simulink model "TrafficLightNegotiationTestBench"  (R2022b)
settings: Solver=ode23tb  StartTime=0.0  StopTime=scenario.StopTime  FixedStep=0.001  RelTol=1e-8  EnableMultiTasking=on
model workspace (MAT data in the model file):
  green = 'green'
values from neighbouring files (symbols this model uses):
  intersectionInfo = evalin('base', 'intersectionInfo')    [HelperTrafficLightNegotiationVisualization.m]
undefined symbols (not defined in the file or in its folder): Curvature, CurvatureDerivative, driving, HeadingAngle, LateralOffset, Left, M, matlabshared, N, referencePathInfo, Right, Strength, Ts, v_set
libraries: drivingscenarioandsensors x4, trackingutilitieslib x1, drivinglib x1
CloseFcn:
  | helperSLTrafficLightNegotiationCleanUp
settings Model: Creator=The MathWorks, Inc.  LastModifiedBy=sangm
settings SolverCC: ZeroCrossAlgorithm=Adaptive  AlgebraicLoopSolver=TrustRegion  PositivePriorityOrder=on  AutoInsertRateTranBlk=on  InsertRTBMode=Always  DecoupledContinuousIntegration=on  MinimalZcImpactIntegration=on  MaxZcPerStep=1
settings DataIOCC: SaveOutput=off  SaveTime=off  ReturnWorkspaceOutputs=off
settings DebuggingCC: MaskedZcDiagnostic=none  IgnoredZcDiagnostic=none  ParameterPrecisionLossMsg=none  UnconnectedInputMsg=warning  UnconnectedOutputMsg=warning  UnconnectedLineMsg=warning  PregeneratedLibrarySubsystemCodeDiagnostic=none  SFMachineParentedDataDiag=warning  ArithmeticOperatorsInVariantConditions=warning
settings HardwareCC: ProdLongLongMode=on
settings ModelReferenceCC: EnableRefExpFcnMdlSchedulingChecks=on
settings SFSimCC: SimUseLocalCustomCode=off
settings RTWCC: GenerateReport=on  RTWUseLocalCustomCode=off  LaunchReport=on  DLArmComputeVersion=19.05
settings ConfigComp: CovScope=ReferencedModels  CovIncludeTopModel=off

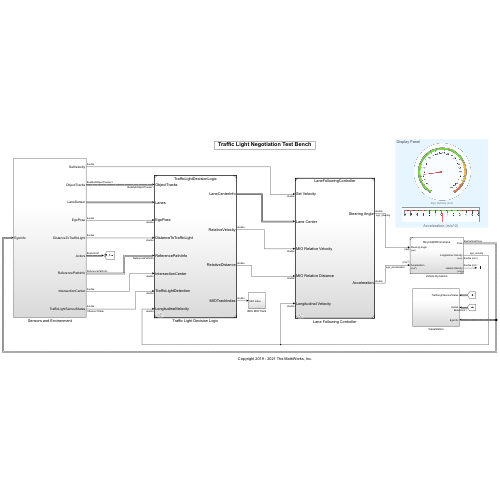
[thumbnail: Simulink's stored preview of the top-level diagram]
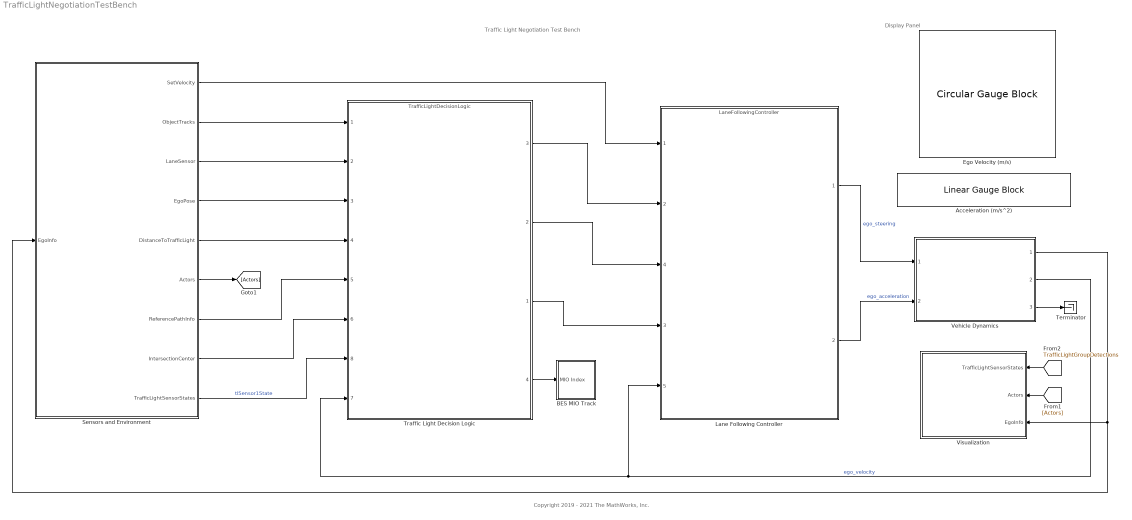
== system TrafficLightNegotiationTestBench ==
  note: Traffic Light Negotiation Test Bench
  note: Display Panel
  note: Copyright 2019 - 2021 The MathWorks, Inc.
  Acceleration (m/s^2) : LinearGaugeBlock  LabelPosition=Hide  ScaleMin=-6  ScaleMax=6
  BES MIO Track : Subsystem
  Ego Velocity (m/s) : CircularGaugeBlock  LabelPosition=Hide  ScaleMax=50
  Lane Following Controller : ModelReference  ModelNameDialog=LaneFollowingController.slx  SimulationMode=Normal  ModelReferenceVersion=6.1
      settings: PortSchema="{\"entries\":[{\"content\":{\"sides\":[{\"content\":{\"connectorIds\":[\"In1\",\"In2\",\"In4\",\"In3\",\"In5\"]},\"type\":\"ConnectorPlacement.EquallySpacedRectSide\",\"uuid\":\"258a64d3-b85d-4414-a7dd-6950fa9dc812\"},{\"content\":{\"connectorIds\":[\"Out1\",\"Out2\"],\"side\":\"RIGHT\"},\"type\":\"ConnectorPlacement.EquallySpacedRectSide\",\"uuid\":\"eccca8be-1d69-4bb6-a162-74a40ef18f77\"},{\"content\":{\"connectorIds\":[],\"side\":\"TOP\"},\"type\":\"ConnectorPlacement.EquallySpacedRectSide\",\"uuid\":\"90abafbb-8c91-4838-b7d8-ed3861625810\"}]},\"type\":\"ConnectorPlacement.EquallySpacedConnector\",\"uuid\":\"818faacf-e725-4a67-9fb9-d6eb3f95c5ad\"}],\"packageUris\":[\"http://schema.mathworks.com/mf0/Connector/R2020b\"],\"version\":\"1.0\"}"
  Sensors and Environment : Subsystem
  Terminator : Terminator
  Traffic Light Decision Logic : ModelReference  ModelNameDialog=TrafficLightDecisionLogic  SimulationMode=Normal  ModelReferenceVersion=5.1
      settings: PortSchema="{\"entries\":[{\"content\":{\"sides\":[{\"content\":{\"connectorIds\":[\"In1\",\"In2\",\"In3\",\"In4\",\"In5\",\"In6\",\"In8\",\"In7\"]},\"type\":\"ConnectorPlacement.EquallySpacedRectSide\",\"uuid\":\"580d7771-a392-489d-ba06-e0a23417c921\"},{\"content\":{\"connectorIds\":[\"Out3\",\"Out2\",\"Out1\",\"Out4\"],\"side\":\"RIGHT\"},\"type\":\"ConnectorPlacement.EquallySpacedRectSide\",\"uuid\":\"34dc41bc-0d5b-42f7-ac4d-a18cefff1604\"},{\"content\":{\"connectorIds\":[],\"side\":\"TOP\"},\"type\":\"ConnectorPlacement.EquallySpacedRectSide\",\"uuid\":\"c461dccf-2cc6-49a6-b643-9bb66a30f56a\"},{\"content\":{\"connectorIds\":[],\"side\":\"HIDDEN\"},\"type\":\"ConnectorPlacement.EquallySpacedRectSide\",\"uuid\":\"944284c5-f0c1-462b-8985-62524d7ec2e9\"}]},\"type\":\"ConnectorPlacement.EquallySpacedConnector\",\"uuid\":\"d6b87f41-7423-4eb9-8350-a9de1b3f3f98\"}],\"packageUris\":[\"http://schema.mathworks.com/mf0/Connector/R2020b\"],\"version\":\"1.0\"}"
  Vehicle Dynamics : Subsystem  ReferencedSubsystem=BicycleWithForceInput
  Visualization : Subsystem
  wires:
  Sensors and Environment/6(Actors) -> [Actors]
  Sensors and Environment/2(ObjectTracks) -> Traffic Light Decision Logic/1
  Lane Following Controller/2 -> Vehicle Dynamics/2  "ego_acceleration"
  Sensors and Environment/1(SetVelocity) -> Lane Following Controller/1
  Vehicle Dynamics/2 -> Traffic Light Decision Logic/7, Lane Following Controller/5  "ego_velocity"
  [TrafficLightGroupDetections] -> Visualization/1(TrafficLightSensorStates)
  Vehicle Dynamics/1 -> Sensors and Environment/1(EgoInfo), Visualization/3(EgoInfo)
  [Actors] -> Visualization/2(Actors)
  Sensors and Environment/4(EgoPose) -> Traffic Light Decision Logic/3
  Sensors and Environment/3(LaneSensor) -> Traffic Light Decision Logic/2
  Sensors and Environment/5(DistanceToTrafficLight) -> Traffic Light Decision Logic/4
  Sensors and Environment/7(ReferencePathInfo) -> Traffic Light Decision Logic/5
  Sensors and Environment/8(IntersectionCenter) -> Traffic Light Decision Logic/6
  Sensors and Environment/9(TrafficLightSensorStates) -> Traffic Light Decision Logic/8  "tlSensor1State"
  Traffic Light Decision Logic/3 -> Lane Following Controller/2
  Traffic Light Decision Logic/1 -> Lane Following Controller/3
  Traffic Light Decision Logic/2 -> Lane Following Controller/4
  Lane Following Controller/1 -> Vehicle Dynamics/1  "ego_steering"
  Traffic Light Decision Logic/4 -> BES MIO Track/1(MIO Index)
  Vehicle Dynamics/3 -> Terminator/1

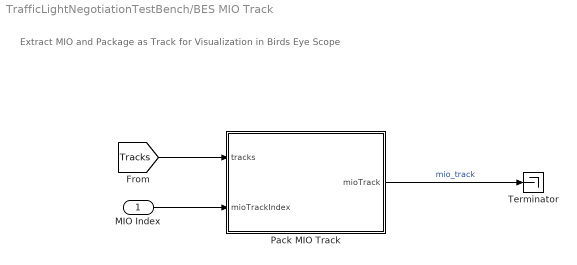
== system TrafficLightNegotiationTestBench/BES MIO Track ==
  note: Extract MIO and Package as Track for Visualization in Birds Eye Scope
  MIO Index : Inport
  Pack MIO Track : MATLAB Function  TreatAsAtomicUnit=on
  Terminator : Terminator
  wires:
  MIO Index/1 -> Pack MIO Track/2(mioTrackIndex)
  [Tracks] -> Pack MIO Track/1(tracks)
  Pack MIO Track/1(mioTrack) -> Terminator/1  "mio_track"

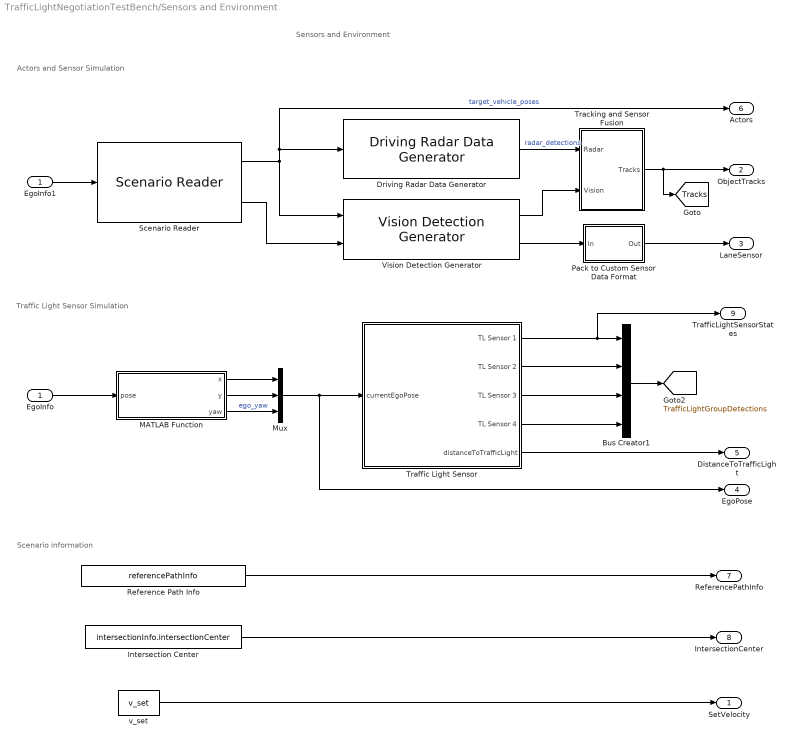
== system TrafficLightNegotiationTestBench/Sensors and Environment ==
  note: Scenario information
  note: Traffic Light Sensor Simulation
  note: Actors and Sensor Simulation
  note: Sensors and Environment
  EgoInfo : Inport
  Bus Creator1 : BusCreator  Inputs=4
  Driving Radar Data Generator : drivingscenarioandsensors/Driving Radar Data Generator  SensorIndex=2  UpdateRate=10  MountingLocation=[ 3.7, 0, 0.2 ]  MountingAngles=[0 0 0]  HasElevation=off  HasRangeRate=on  HasNoise=on  HasFalseAlarms=on  HasOcclusion=on  MaxNumReportsSource=Property  MaxNumReports=50  TargetReportFormat=Clustered detections  DetectionCoordinates=Body  TrackCoordinates=Body  BusNameSource=Property  BusName=BusRadar  AzimuthResolution=4  ElevationResolution=5  RangeResolution=2.5  RangeRateResolution=0.5  AzimuthBiasFraction=0.1  ElevationBiasFraction=0.1  RangeBiasFraction=0.05  RangeRateBiasFraction=0.05  FieldOfView=[ 20, 5 ]  RangeLimits=[ 0, 174 ]  RangeRateLimits=[ -100, 100 ]  DetectionProbability=0.9  FalseAlarmRate=1e-06  ReferenceRange=100  ReferenceRCS=0  CenterFrequency=77e9  FilterInitializationFcn=initcvekf  ConfirmationThreshold=[2 3]  DeletionThreshold=[5 5]  InitialSeedSource=Repeatable  InitialSeed=0  UsedSeed=matlabshared.tracking.internal.SimulinkUtilities.seedManager(gcb)  ProfilesSource=From Scenario Reader block  ProfilesParameters=driving.internal.ActorProfilesRadarParameters  ProfilesExpression=struct('ClassID',0,'Length',4.7,'Width',1.8,'Height',1.4,'OriginOffset',[-1.35 0 0],'RCSPattern',[10 10;10 10],'RCSAzimuthAngles',[-180 180],'RCSElevationAngles',[-90 90])
  EgoInfo1 : InportShadow
  Intersection Center : Constant  Value=intersectionInfo.intersectionCenter  SampleTime=Ts
      settings: AttributesFormatString=|
      | ------------------------------
      |    Value = %<Value>
  MATLAB Function : MATLAB Function  TreatAsAtomicUnit=on
  Mux : Mux  Inputs=3
  Pack to Custom Sensor Data Format : Subsystem
  Reference Path Info : Constant  Value=referencePathInfo  OutDataTypeStr=Bus: ReferencePathInfo  SampleTime=Ts
      settings: AttributesFormatString=|
      | --------------------------
      |   Value = %<Value>
  Scenario Reader : drivingscenarioandsensors/Scenario Reader  ScenarioSource=From workspace  ScenarioFileName=EgoVehicleGoesStraight.mat  ScenarioVariableName=scenario  OutputCoordinateSystem=Vehicle coordinates  EgoVehicleSource=Input port  EgoVehicleActorID=egoVehicle.ActorID  OrientVehiclesOnRoad=on  OutputEgoVehiclePose=off  OutputEgoVehicleState=off  SampleTime=Ts  LaneBoundaryOutput=All lane boundaries  LaneBoundaryDistance=0:0.5:60  LaneBoundaryLocation=Center of lane markings  BusNameSource=Auto  BusName=BusActors  BusNumActorsSource=Scenario  BusNumActors=100  BusName2Source=Auto  BusName2=BusLaneBoundaries  BusNumLaneBoundariesSource=Scenario  BusNumLaneBoundaries=10  BusName3Source=Auto  BusName3=BusEgoActor  BusName4Source=Auto  BusName4=BusEgoState  ShowCoordinateLabels=on  SimulateUsing=Interpreted execution
  Tracking and Sensor Fusion : Subsystem  TreatAsAtomicUnit=on  SystemSampleTime=Ts
      settings: RTWFileNameOpts=Use function name
  Traffic Light Sensor : Subsystem  mask{TrafficLightSensorModeSelection=Cycle, TrafficLightPosition=intersectionInfo.tlSensor1Position}
      mask prompts: TrafficLightSensorModeSelection "Traffic Light Sensor Mode:"; TrafficLightPosition "Traffic Light Position:"
      mask TypeOptions TrafficLightSensorModeSelection: Steady Green | Steady Red | Cycle
      mask TypeOptions TrafficLightPosition: TrafficLightPosition/Value
      mask DialogControl DescTextVar Prompt: Simulate a traffic light sensor.
  Vision Detection Generator : drivingscenarioandsensors/Vision Detection Generator  SensorIndex=1  DetectorOutput=Lanes and objects  UpdateInterval=0.1  LaneUpdateInterval=0.1  SensorLocation=[ 1.9, 0 ]  Height=1.1  Yaw=0  Pitch=1  Roll=0  BusNameSource=Property  BusName=BusVision  BusName2Source=Property  BusName2=BusLanes  MaxNumDetectionsSource=Property  MaxNumDetections=20  MaxNumLanesSource=Property  MaxNumLanes=2  DetectionCoordinates=Ego Cartesian  SimulateUsing=Interpreted execution  MaxRange=150  BoundingBoxAccuracy=5  ProcessNoiseIntensity=5  MaxSpeed=50  MaxAllowedOcclusion=0.5  MinObjectImageSize=[ 10, 10 ]  DetectionProbability=1  FalsePositivesPerImage=0  MinLaneImageSize=[ 20, 3 ]  LaneBoundaryAccuracy=3  HasNoise=off  InitialSeedSource=Repeatable  InitialSeed=0  UsedSeed=driving.internal.SimulinkUtilities.seedManager(gcb)  ActorProfilesSource=From Scenario Reader block  ActorProfilesParameters=driving.internal.ActorProfilesParameters  ActorProfilesExpression=struct( 'ClassID', 0, 'Length', 4.7, 'Width', 1.8, 'Height', 1.4, 'OriginOffset', [ -1.35, 0, 0 ] )  Intrinsics=driving.internal.cameraIntrinsics('FocalLength',[ 800,800 ])
  v_set : Constant  Value=v_set
  SetVelocity : Outport
  ObjectTracks : Outport  Port=2
  LaneSensor : Outport  Port=3  VectorParamsAs1DForOutWhenUnconnected=off
  EgoPose : Outport  Port=4
  DistanceToTrafficLight : Outport  Port=5
  Actors : Outport  Port=6
  ReferencePathInfo : Outport  Port=7
  IntersectionCenter : Outport  Port=8
  TrafficLightSensorStates : Outport  Port=9
  tag scope: Tracks=global, TrafficLightGroupDetections=global
  wires:
  Vision Detection Generator/2 -> Pack to Custom Sensor Data Format/1(In)
  Pack to Custom Sensor Data Format/1(Out) -> LaneSensor/1
  Scenario Reader/2 -> Vision Detection Generator/2
  Vision Detection Generator/1 -> Tracking and Sensor Fusion/2(Vision)
  Driving Radar Data Generator/1 -> Tracking and Sensor Fusion/1(Radar)  "radar_detections"
  EgoInfo/1 -> MATLAB Function/1(pose)
  MATLAB Function/3(yaw) -> Mux/3  "ego_yaw"
  MATLAB Function/2(y) -> Mux/2
  MATLAB Function/1(x) -> Mux/1
  Mux/1 -> EgoPose/1, Traffic Light Sensor/1(currentEgoPose)
  Tracking and Sensor Fusion/1(Tracks) -> [Tracks], ObjectTracks/1
  Scenario Reader/1 -> Driving Radar Data Generator/1, Actors/1, Vision Detection Generator/1  "target_vehicle_poses"
  EgoInfo1/1 -> Scenario Reader/1
  Traffic Light Sensor/5(distanceToTrafficLight) -> DistanceToTrafficLight/1
  Reference Path Info/1 -> ReferencePathInfo/1
  v_set/1 -> SetVelocity/1
  Intersection Center/1 -> IntersectionCenter/1
  Traffic Light Sensor/1(TL Sensor 1) -> TrafficLightSensorStates/1, Bus Creator1/1
  Traffic Light Sensor/2(TL Sensor 2) -> Bus Creator1/2
  Traffic Light Sensor/3(TL Sensor 3) -> Bus Creator1/3
  Traffic Light Sensor/4(TL Sensor 4) -> Bus Creator1/4
  Bus Creator1/1 -> [TrafficLightGroupDetections]

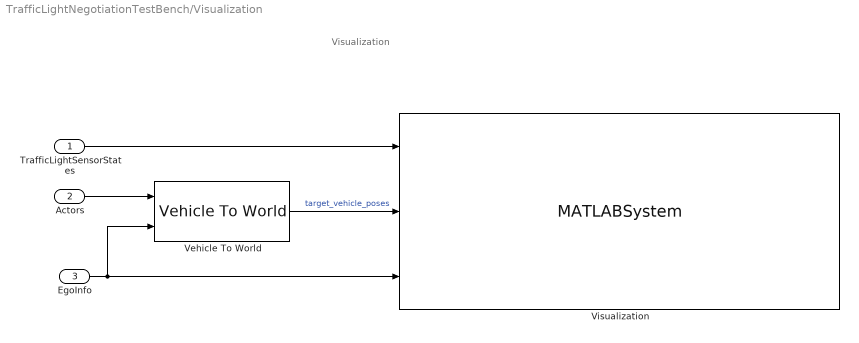
== system TrafficLightNegotiationTestBench/Visualization ==
  note: Visualization
  TrafficLightSensorStates : Inport
  Actors : Inport  Port=2
  EgoInfo : Inport  Port=3
  Vehicle To World : drivingscenarioandsensors/Vehicle To World  BusNameSource=Auto  BusName=BusVehicleToWorldActors  SimulateUsing=Interpreted execution
  Visualization : MATLABSystem  System=HelperTrafficLightNegotiationVisualization
      mask Type: HelperTrafficLightNegotiationVisualization
      mask Display:
      | disp('HelperTrafficLightNegotiationVisualization');
      | port_label('input',1,'TrafficLightSensorStates');
      | port_label('input',2,'TargetPoses');
      | port_label('input',3,'EgoInfo');
  wires:
  TrafficLightSensorStates/1 -> Visualization/1
  Actors/1 -> Vehicle To World/1
  EgoInfo/1 -> Vehicle To World/2, Visualization/3
  Vehicle To World/1 -> Visualization/2  "target_vehicle_poses"

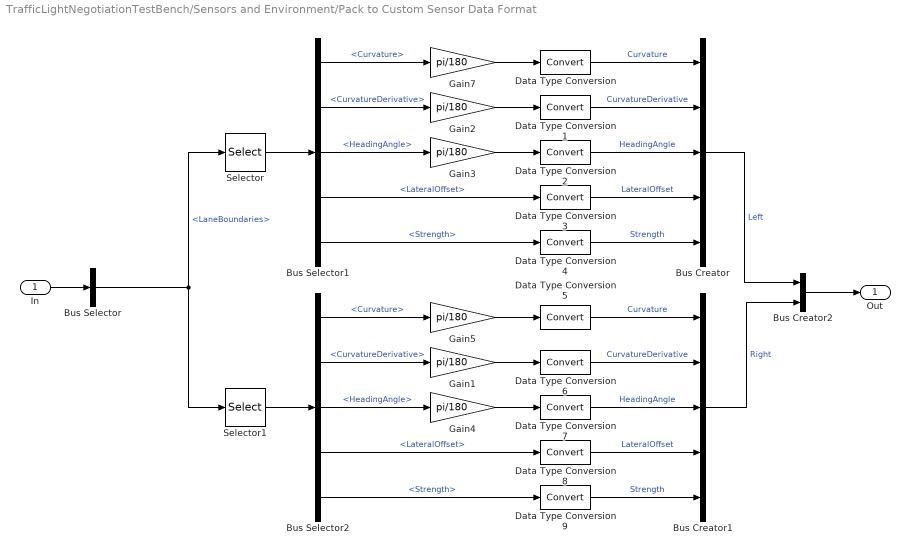
== system TrafficLightNegotiationTestBench/Sensors and Environment/Pack to Custom Sensor Data Format ==
  In : Inport
  Bus Creator : BusCreator  Inputs=Curvature,CurvatureDerivative,HeadingAngle,LateralOffset,Strength  OutDataTypeStr=Bus: LaneSensorBoundaries
  Bus Creator1 : BusCreator  Inputs=Curvature,CurvatureDerivative,HeadingAngle,LateralOffset,Strength  OutDataTypeStr=Bus: LaneSensorBoundaries
  Bus Creator2 : BusCreator  Inputs=Left,Right  OutDataTypeStr=Bus: LaneSensor
  Bus Selector : BusSelector  OutputSignals=LaneBoundaries
  Bus Selector1 : BusSelector  OutputSignals=Curvature,CurvatureDerivative,HeadingAngle,LateralOffset,Strength
  Bus Selector2 : BusSelector  OutputSignals=Curvature,CurvatureDerivative,HeadingAngle,LateralOffset,Strength
  Data Type Conversion{,1..9} (10 alike) : DataTypeConversion  SaturateOnIntegerOverflow=off  RndMeth=Floor
  Gain{1..5,7} (6 alike) : Gain  Gain=pi/180
  Selector : Selector  InputPortWidth=2  IndexOptions=Index vector (dialog)  Indices=1  OutputSizes=1
  Selector1 : Selector  InputPortWidth=2  IndexOptions=Index vector (dialog)  Indices=2  OutputSizes=1
  Out : Outport  VectorParamsAs1DForOutWhenUnconnected=off
  wires:
  In/1 -> Bus Selector/1
  Bus Selector/1 -> Selector/1, Selector1/1  "<LaneBoundaries>"
  Selector/1 -> Bus Selector1/1
  Bus Selector1/2 -> Gain2/1  "<CurvatureDerivative>"
  Bus Selector1/1 -> Gain7/1  "<Curvature>"
  Bus Selector1/3 -> Gain3/1  "<HeadingAngle>"
  Gain7/1 -> Data Type Conversion/1
  Gain2/1 -> Data Type Conversion1/1
  Gain3/1 -> Data Type Conversion2/1
  Bus Selector1/4 -> Data Type Conversion3/1  "<LateralOffset>"
  Bus Selector1/5 -> Data Type Conversion4/1  "<Strength>"
  Data Type Conversion/1 -> Bus Creator/1  "Curvature"
  Data Type Conversion1/1 -> Bus Creator/2  "CurvatureDerivative"
  Data Type Conversion2/1 -> Bus Creator/3  "HeadingAngle"
  Data Type Conversion3/1 -> Bus Creator/4  "LateralOffset"
  Data Type Conversion4/1 -> Bus Creator/5  "Strength"
  Data Type Conversion9/1 -> Bus Creator1/5  "Strength"
  Data Type Conversion6/1 -> Bus Creator1/2  "CurvatureDerivative"
  Data Type Conversion7/1 -> Bus Creator1/3  "HeadingAngle"
  Data Type Conversion8/1 -> Bus Creator1/4  "LateralOffset"
  Data Type Conversion5/1 -> Bus Creator1/1  "Curvature"
  Bus Selector2/1 -> Gain5/1  "<Curvature>"
  Selector1/1 -> Bus Selector2/1
  Bus Selector2/4 -> Data Type Conversion8/1  "<LateralOffset>"
  Bus Selector2/5 -> Data Type Conversion9/1  "<Strength>"
  Bus Selector2/2 -> Gain1/1  "<CurvatureDerivative>"
  Gain4/1 -> Data Type Conversion7/1
  Gain5/1 -> Data Type Conversion5/1
  Gain1/1 -> Data Type Conversion6/1
  Bus Selector2/3 -> Gain4/1  "<HeadingAngle>"
  Bus Creator2/1 -> Out/1
  Bus Creator/1 -> Bus Creator2/1  "Left"
  Bus Creator1/1 -> Bus Creator2/2  "Right"

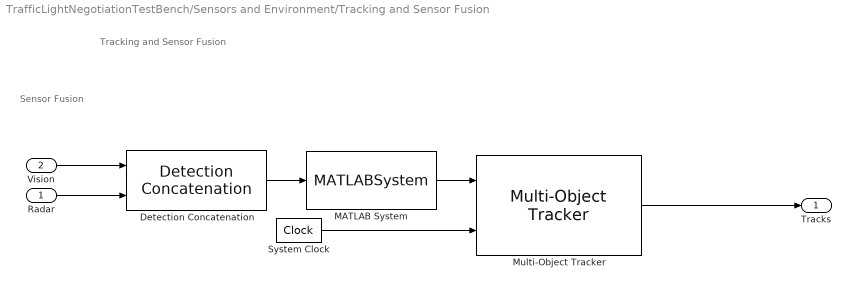
== system TrafficLightNegotiationTestBench/Sensors and Environment/Tracking and Sensor Fusion ==
  note: Tracking and Sensor Fusion
  note: Sensor Fusion
  Radar : Inport  PortDimensions=[1 1]  BusOutputAsStruct=on
  Vision : Inport  Port=2  PortDimensions=[1 1]  BusOutputAsStruct=on
  Detection Concatenation : trackingutilitieslib/Detection Concatenation  NumInputs=2  BusNameSource=Auto  BusName=BusDetectionConcatenation1  SimulateUsing=Interpreted execution
  MATLAB System : MATLABSystem  System=helperVehicleSize  VehicleSize=vehicleLength  BusNameSource=Auto  BusName=BusVehicleSizeDetections  SimulateUsing=Interpreted execution
      mask Type: helperVehicleSize
      mask Display:
      | disp('helperVehicleSize');
      | port_label('input',1,'In');
      | port_label('output',1,'Out');
  Multi-Object Tracker : drivinglib/Multi-Object Tracker  TrackerIndex=uint32( 0 )  FilterInitializationFcn=initcvekf  AssignmentThreshold=assignThresh  ConfirmationThreshold=[ M, N ]  DeletionThreshold=[ 5, 5 ]  MaxNumTracks=numTracks  MaxNumSensors=numSensors  OOSMHandling=Terminate  StateParametersSimulink=struct  HasStateParametersInput=off  TimeInputSource=Input port  HasCostMatrixInput=off  HasDetectableTrackIDsInput=off  BusNameSource=Property  BusName=BusMultiObjectTracker1  TentativeTracksOutputPort=off  AllTracksOutputPort=off  SimulateUsing=Interpreted execution
  System Clock : DigitalClock  SampleTime=-1
  Tracks : Outport  PortDimensions=[1 1]  VectorParamsAs1DForOutWhenUnconnected=off  BusOutputAsStruct=on
  wires:
  System Clock/1 -> Multi-Object Tracker/2
  Vision/1 -> Detection Concatenation/1
  Radar/1 -> Detection Concatenation/2
  Multi-Object Tracker/1 -> Tracks/1
  Detection Concatenation/1 -> MATLAB System/1
  MATLAB System/1 -> Multi-Object Tracker/1

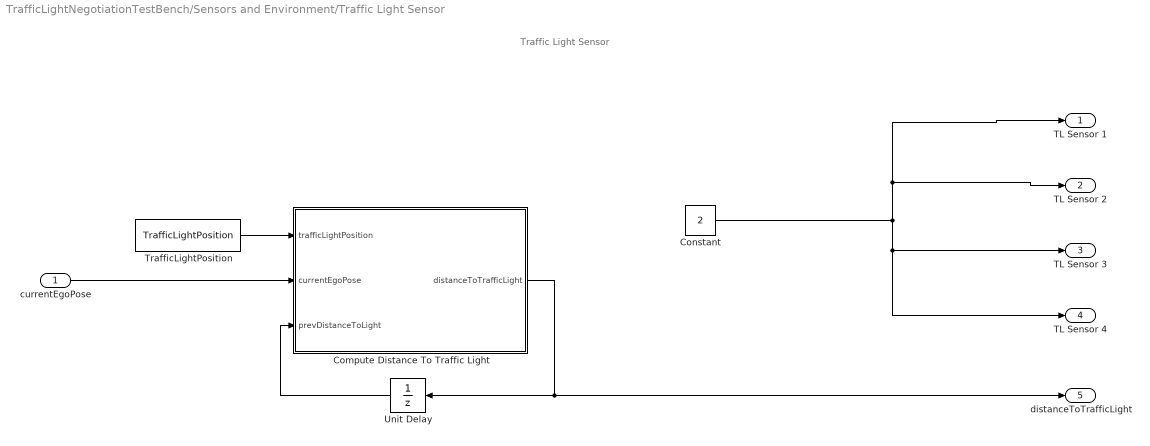
== system TrafficLightNegotiationTestBench/Sensors and Environment/Traffic Light Sensor ==
  note: Traffic Light Sensor
  currentEgoPose : Inport
  Compute Distance To Traffic Light : MATLAB Function  TreatAsAtomicUnit=on  mask{minTLDist=3}
      mask prompts: minTLDist "Minimum distance to traffic light"
  Constant : Constant  Value=2  OutDataTypeStr=double
  TrafficLightPosition : Constant  Value=TrafficLightPosition
  Unit Delay : UnitDelay  InitialCondition=100  SampleTime=-1  HasFrameUpgradeWarning=on
  TL Sensor 1 : Outport
  TL Sensor 2 : Outport  Port=2
  TL Sensor 3 : Outport  Port=3
  TL Sensor 4 : Outport  Port=4
  distanceToTrafficLight : Outport  Port=5
  wires:
  TrafficLightPosition/1 -> Compute Distance To Traffic Light/1(trafficLightPosition)
  Unit Delay/1 -> Compute Distance To Traffic Light/3(prevDistanceToLight)
  currentEgoPose/1 -> Compute Distance To Traffic Light/2(currentEgoPose)
  Constant/1 -> TL Sensor 2/1, TL Sensor 1/1, TL Sensor 4/1, TL Sensor 3/1
  Compute Distance To Traffic Light/1(distanceToTrafficLight) -> distanceToTrafficLight/1, Unit Delay/1

== matlab function TrafficLightNegotiationTestBench/BES MIO Track/Pack MIO Track ==
  data: tracks input; mioTrack output Bus: BusMultiObjectTracker1; mioTrackIndex input
function mioTrack = fcn(tracks, mioTrackIndex)
% Extract MIO track and package for visualization in Birds Eye Scope

mioTrack = tracks;

if mioTrackIndex > 0
    % First track represents MIO
    mioTrack.NumTracks = 1;
    mioTrack.Tracks(1) = tracks.Tracks(mioTrackIndex);
else
    % No valid MIO track
    mioTrack.NumTracks = 0;
end

== matlab function TrafficLightNegotiationTestBench/Sensors and Environment/MATLAB Function ==
  data: pose input; x output; y output; yaw output
function [x, y, yaw] = poseToSim(pose)

pos_Rr = pose.Position([1,2])';
theta = pose.Yaw;

pos_Cen = pos_Rr+[cosd(theta) sind(theta)]';

x = pos_Cen(1);
y = pos_Cen(2);
yaw = pose.Yaw;

== matlab function TrafficLightNegotiationTestBench/Sensors and Environment/Traffic Light Sensor/Compute Distance To Traffic Light ==
  data: trafficLightPosition input; currentEgoPose input; prevDistanceToLight input; distanceToTrafficLight output; minTLDist parameter
function distanceToTrafficLight   = computeDistanceToTrafficLight(trafficLightPosition, currentEgoPose, prevDistanceToLight, minTLDist)

%computeDistanceToTrafficLight Compute distance to upcoming traffic light.

distanceToTrafficLight = ...
    helperSLComputeDistanceToTrafficLight(trafficLightPosition, ...
    currentEgoPose, prevDistanceToLight, minTLDist);
